simulink subsystem "Aerodyn"  (R2020b)
settings: Solver=VariableStepAuto  StartTime=0.0  StopTime=10.0  RelTol=1e-3
undefined symbols (not defined in the file): Aerodynamics
settings Model: Creator=NicolasS  LastModifiedBy=adith

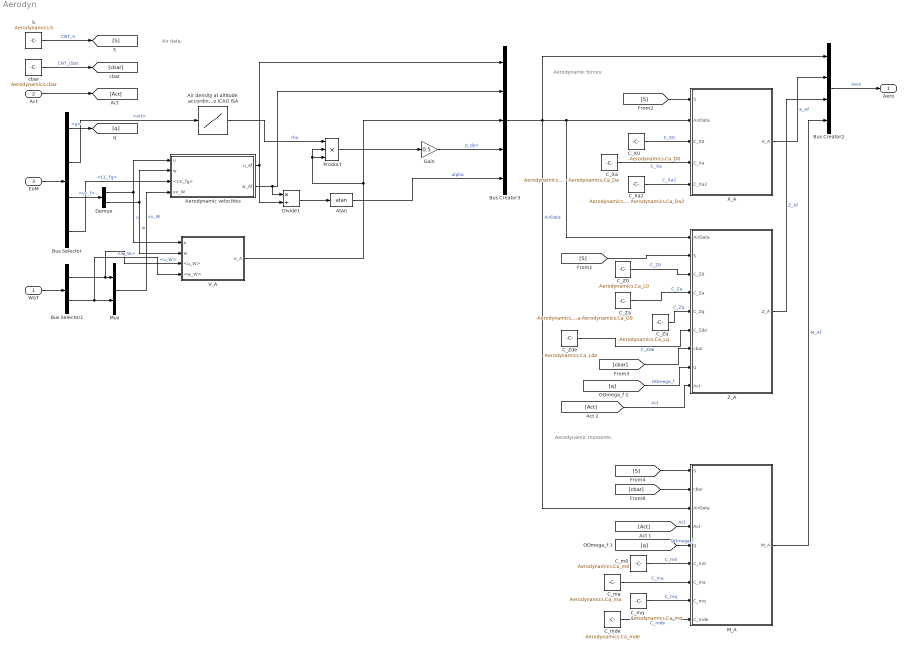
== system Aerodyn ==
  note: Air data:
  note: Aerodynamic moments:
  note: Aerodynamic forces:
  WaT : Inport  OutDataTypeStr=Bus: WaT
  Act : Inport  Port=2  OutDataTypeStr=Bus: Act
  EoM : Inport  Port=3  OutDataTypeStr=Bus: EoM
  Aerodynamic velocities : Subsystem
  Air density at altitude according to ICAO ISA : Lookup_n-D  NumberOfTableDimensions=1  BreakpointsForDimension1=Aerodynamics.LUT_Alt  Table=Aerodynamics.LUT_rho  ExtrapMethod=Clip  InternalRulePriority=Speed  RndMeth=Simplest  InputSameDT=on
  Atan : Trigonometry  Operator=atan
  Bus Creator2 : BusCreator  Inputs=4  OutDataTypeStr=Bus: Aero
  Bus Creator3 : BusCreator  Inputs=5  OutDataTypeStr=Bus: AirData
  Bus Selector : BusSelector  OutputSignals=q,Alt,vv_f,CC.CC_fg
  Bus Selector1 : BusSelector  OutputSignals=u_W,w_W
  C_X0 : Constant  Value=-Aerodynamics.Ca_D0  VectorParams1D=off  OutDataTypeStr=double  SampleTime=-1
  C_Xa : Constant  Value=Aerodynamics.Ca_L0 - Aerodynamics.Ca_Da  VectorParams1D=off  OutDataTypeStr=double  SampleTime=-1
  C_Xa2 : Constant  Value=Aerodynamics.Ca_La - Aerodynamics.Ca_Da2  VectorParams1D=off  OutDataTypeStr=double  SampleTime=-1
  C_Z0 : Constant  Value=-Aerodynamics.Ca_L0  VectorParams1D=off  OutDataTypeStr=double  SampleTime=-1
  C_Za : Constant  Value=-Aerodynamics.Ca_La-Aerodynamics.Ca_D0  VectorParams1D=off  OutDataTypeStr=double  SampleTime=-1
  C_Zde : Constant  Value=-Aerodynamics.Ca_Lde  VectorParams1D=off  OutDataTypeStr=double  SampleTime=-1
  C_Zq : Constant  Value=-Aerodynamics.Ca_Lq  VectorParams1D=off  OutDataTypeStr=double  SampleTime=-1
  C_m0 : Constant  Value=Aerodynamics.Ca_m0  VectorParams1D=off  OutDataTypeStr=double  SampleTime=-1
  C_ma : Constant  Value=Aerodynamics.Ca_ma  VectorParams1D=off  OutDataTypeStr=double  SampleTime=-1
  C_mde : Constant  Value=Aerodynamics.Ca_mde  VectorParams1D=off  OutDataTypeStr=double  SampleTime=-1
  C_mq : Constant  Value=Aerodynamics.Ca_mq  VectorParams1D=off  OutDataTypeStr=double  SampleTime=-1
  Demux : Demux  Outputs=2
  Divide1 : Product  Inputs=*/
  Gain : Gain  Gain=0.5
  M_A : MATLAB Function  TreatAsAtomicUnit=on
  Mux : Mux  Inputs=2
  Product : Product  Inputs=3
  S : Constant  Value=Aerodynamics.S  OutDataTypeStr=double  SampleTime=-1
  V_A : Subsystem
  X_A : MATLAB Function  TreatAsAtomicUnit=on
  Z_A : MATLAB Function  TreatAsAtomicUnit=on
  cbar : Constant  Value=Aerodynamics.cbar  OutDataTypeStr=double  SampleTime=-1
  Aero : Outport  OutDataTypeStr=Bus: Aero
  wires:
  Act/1 -> [Act]
  C_m0/1 -> M_A/6(C_m0)  "C_m0"
  C_mq/1 -> M_A/8(C_mq)  "C_mq"
  C_ma/1 -> M_A/7(C_ma)  "C_ma"
  C_Xa/1 -> X_A/4(C_Xa)  "C_Xa"
  C_Xa2/1 -> X_A/5(C_Xa2)  "C_Xa2"
  S/1 -> [S]  "CNT_S"
  Bus Creator2/1 -> Aero/1  "Aero"
  C_mde/1 -> M_A/9(C_mde)  "C_mde"
  C_X0/1 -> X_A/3(C_X0)  "C_X0"
  Bus Creator3/1 -> Bus Creator2/1, M_A/3(AirData), Z_A/1(AirData), X_A/2(AirData)  "AirData"
  Bus Selector/2 -> Air density at altitude according to ICAO ISA/1  "<Alt>"
  Atan/1 -> Bus Creator3/5  "alpha"
  EoM/1 -> Bus Selector/1
  Bus Selector/1 -> [q]  "<q>"
  WaT/1 -> Bus Selector1/1
  Bus Selector1/1 -> Mux/1, V_A/3(<u_W>)  "<u_W>"
  Bus Selector1/2 -> Mux/2, V_A/4(<w_W>)  "<w_W>"
  cbar/1 -> [cbar]  "CNT_cbar"
  [S] -> X_A/1(S)
  [S] -> M_A/1(S)
  [cbar] -> M_A/2(cbar)
  [Act] -> M_A/4(Act)  "Act"
  [q] -> M_A/5(q)  "OOmega_f"
  X_A/1(X_A) -> Bus Creator2/2  "X_Af"
  Z_A/1(Z_A) -> Bus Creator2/3  "Z_Af"
  M_A/1(M_A) -> Bus Creator2/4  "M_Af"
  Bus Selector/3 -> Demux/1  "<vv_f>"
  Demux/2 -> Aerodynamic velocities/2(w), V_A/2(w)  "w"
  Demux/1 -> Aerodynamic velocities/1(u), V_A/1(u)  "u"
  [S] -> Z_A/2(S)
  C_Z0/1 -> Z_A/3(C_Z0)  "C_Z0"
  C_Za/1 -> Z_A/4(C_Za)  "C_Za"
  [cbar] -> Z_A/7(cbar)
  [q] -> Z_A/8(q)  "OOmega_f"
  C_Zq/1 -> Z_A/5(C_Zq)  "C_Zq"
  C_Zde/1 -> Z_A/6(C_Zde)  "C_Zde"
  [Act] -> Z_A/9(Act)  "Act"
  Air density at altitude according to ICAO ISA/1 -> Product/1  "rho"
  Gain/1 -> Bus Creator3/4  "p_dyn"
  Product/1 -> Gain/1
  Divide1/1 -> Atan/1
  Aerodynamic velocities/2(w_Af) -> Bus Creator3/2, Divide1/1
  Aerodynamic velocities/1(u_Af) -> Divide1/2, Bus Creator3/1
  Bus Selector/4 -> Aerodynamic velocities/3(<CC_fg>)  "<CC_fg>"
  Mux/1 -> Aerodynamic velocities/4(vv_W)  "vv_W"
  V_A/1(V_A) -> Product/2, Product/3, Bus Creator3/3

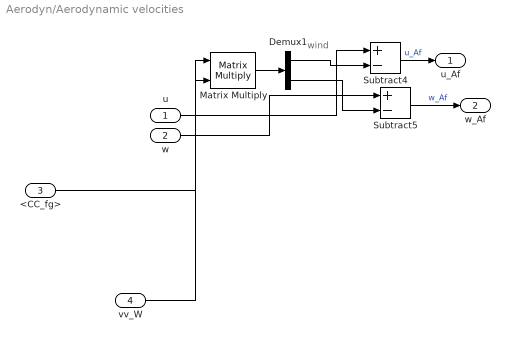
== system Aerodyn/Aerodynamic velocities ==
  note: wind
  u : Inport
  w : Inport  Port=2
  <CC_fg> : Inport  Port=3
  vv_W : Inport  Port=4
  Demux1 : Demux  Outputs=2
  Matrix Multiply : Product  Multiplication=Matrix(*)
  Subtract4 : Sum  Inputs=+-
  Subtract5 : Sum  Inputs=+-
  u_Af : Outport
  w_Af : Outport  Port=2
  wires:
  w/1 -> Subtract5/1
  vv_W/1 -> Matrix Multiply/2
  Demux1/1 -> Subtract4/2
  u/1 -> Subtract4/1
  Demux1/2 -> Subtract5/2
  Subtract5/1 -> w_Af/1  "w_Af"
  <CC_fg>/1 -> Matrix Multiply/1
  Matrix Multiply/1 -> Demux1/1
  Subtract4/1 -> u_Af/1  "u_Af"

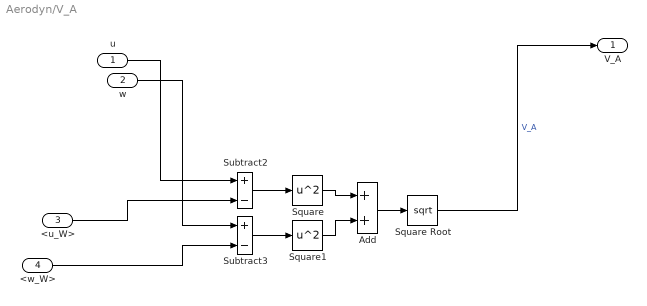
== system Aerodyn/V_A ==
  u : Inport
  w : Inport  Port=2
  <u_W> : Inport  Port=3
  <w_W> : Inport  Port=4
  Add : Sum
  Square : Math  Operator=square  SaturateOnIntegerOverflow=on
  Square Root : Sqrt  SaturateOnIntegerOverflow=on
  Square1 : Math  Operator=square  SaturateOnIntegerOverflow=on
  Subtract2 : Sum  Inputs=+-
  Subtract3 : Sum  Inputs=+-
  V_A : Outport
  wires:
  Square Root/1 -> V_A/1  "V_A"
  u/1 -> Subtract2/1
  Square1/1 -> Add/2
  Subtract3/1 -> Square1/1
  Square/1 -> Add/1
  <u_W>/1 -> Subtract2/2
  Subtract2/1 -> Square/1
  Add/1 -> Square Root/1
  w/1 -> Subtract3/1
  <w_W>/1 -> Subtract3/2

== matlab function Aerodyn/Z_A ==
  data: AirData input; S input; Z_A output; C_Z0 input; C_Za input; C_Zq input; C_Zde input; cbar input; q input; Act input

%%%%%%%%%%%%%%%%%%%%%%
% Body-fixed Z force %
%%%%%%%%%%%%%%%%%%%%%%

function Z_A = fcn(AirData,S,C_Z0,C_Za,C_Zq,C_Zde,cbar,q,Act)

Z_A = AirData.p_dyn*S*(C_Z0 + (C_Za*AirData.alpha) + (C_Zq*(cbar/AirData.V_A)*q) + (C_Zde*Act.de) ) ;

== matlab function Aerodyn/M_A ==
  data: S input; cbar input; AirData input Bus: AirData size=1; Act input; q input; C_m0 input; C_ma input; C_mq input; C_mde input; M_A output

%%%%%%%%%%%%%%%%%%%%%%%%%%%
% Body-fixed pitch moment %
%%%%%%%%%%%%%%%%%%%%%%%%%%%

function M_A = fcn(S,cbar,AirData,Act,q,C_m0,C_ma,C_mq,C_mde)

M_A = AirData.p_dyn*S*cbar*(C_m0+ (C_ma*AirData.alpha) + (C_mq*(cbar/AirData.V_A)*q)+ (C_mde*Act.de));

== matlab function Aerodyn/X_A ==
  data: S input; AirData input Bus: AirData size=1; C_X0 input; C_Xa input; C_Xa2 input; X_A output

%%%%%%%%%%%%%%%%%%%%%%
% Body-fixed X force %
%%%%%%%%%%%%%%%%%%%%%%

function X_A = fcn(S,AirData,C_X0,C_Xa,C_Xa2)

X_A = AirData.p_dyn*S*(C_X0 +(C_Xa*AirData.alpha) +(C_Xa2*AirData.alpha*AirData.alpha)) ;
